simulink model "QuadCopter_Blocks"  (R2014b)
settings: Solver=ode45  StartTime=0.0  StopTime=10.0  RelTol=1e-3
settings Model: Creator=Samy.Amin  LastModifiedBy=Samy.Amin

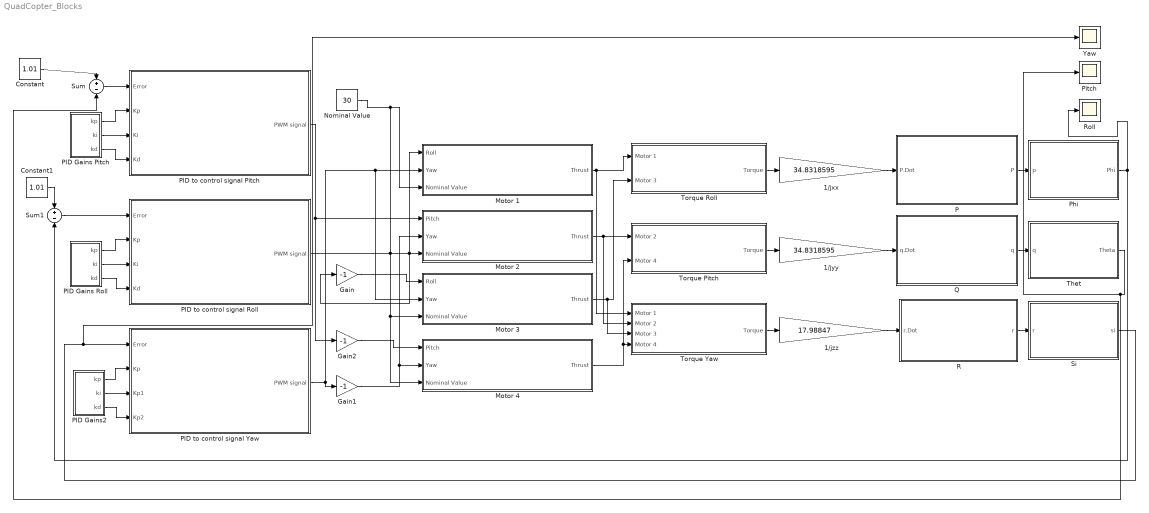
== system QuadCopter_Blocks ==
  1/jxx : Gain  Gain=34.8318595
  1/jyy : Gain  Gain=34.8318595
  1/jzz : Gain  Gain=17.98847
  Constant : Constant  Value=1.01
  Constant1 : Constant  Value=1.01
  Gain : Gain  Gain=-1
  Gain1 : Gain  Gain=-1
  Gain2 : Gain  Gain=-1
  Motor 1 : Subsystem
  Motor 2 : Subsystem
  Motor 3 : Subsystem
  Motor 4 : Subsystem
  Nominal Value : Constant  Value=30
  "P " : Subsystem
  PID Gains Pitch : Subsystem
  PID Gains Roll : Subsystem
  PID Gains2 : Subsystem
  "PID to control signal Pitch " : Subsystem
  PID to control signal Roll : Subsystem
  PID to control signal Yaw : Subsystem
  Phi : Subsystem
  Pitch : Scope
  Q : Subsystem
  R : Subsystem
  Roll : Scope
  Si : Subsystem
  Sum : Sum  Inputs=+-
  Sum1 : Sum  Inputs=+-
  Thet : Subsystem
  Torque Pitch : Subsystem
  Torque Roll : Subsystem
  Torque Yaw : Subsystem
  Yaw : Scope
      settings: SaveName=ScopeData2
  wires:
  "PID to control signal Pitch "/1("PWM signal ") -> Motor 2/1(Pitch), Gain2/1
  Gain2/1 -> Motor 4/1(Pitch)
  PID to control signal Roll/1("PWM signal ") -> Motor 1/1(Roll), Gain/1
  Gain/1 -> Motor 3/1(Roll)
  PID to control signal Yaw/1("PWM signal ") -> Gain1/1, Motor 3/2(Yaw), Motor 1/2(Yaw)
  Gain1/1 -> Motor 4/2(Yaw), Motor 2/2(Yaw)
  Nominal Value/1 -> Motor 4/3(Nominal Value), Motor 3/3(Nominal Value), Motor 2/3(Nominal Value), Motor 1/3(Nominal Value)
  Motor 1/1(Thrust) -> Torque Yaw/1(Motor 1), Torque Roll/1(Motor 1)
  Motor 3/1(Thrust) -> Torque Yaw/3(Motor 3), Torque Roll/2(Motor 3)
  Motor 2/1(Thrust) -> Torque Yaw/2("Motor 2 "), Torque Pitch/1(Motor 2)
  Motor 4/1(Thrust) -> Torque Yaw/4(Motor 4), Torque Pitch/2(Motor 4)
  Torque Roll/1(Torque) -> 1/jxx/1
  Torque Pitch/1(Torque) -> 1/jyy/1
  1/jxx/1 -> "P "/1(P.Dot)
  1/jyy/1 -> Q/1(q.Dot)
  "P "/1(P) -> Phi/1(p)
  Q/1(q) -> Thet/1(q)
  Phi/1(Phi) -> Roll/1, Sum1/2
  Thet/1(Theta) -> Sum/2, Pitch/1
  PID Gains Pitch/1(kp) -> "PID to control signal Pitch "/2(Kp)
  PID Gains Pitch/2(ki) -> "PID to control signal Pitch "/3(Ki)
  PID Gains Pitch/3(kd) -> "PID to control signal Pitch "/4(Kd)
  PID Gains Roll/1(kp) -> PID to control signal Roll/2(Kp)
  PID Gains Roll/2(ki) -> PID to control signal Roll/3(Ki)
  PID Gains Roll/3(kd) -> PID to control signal Roll/4(Kd)
  PID Gains2/1(kp) -> PID to control signal Yaw/2(Kp)
  PID Gains2/2(ki) -> PID to control signal Yaw/3(Kp1)
  PID Gains2/3(kd) -> PID to control signal Yaw/4(Kp2)
  Si/1(si) -> Yaw/1, PID to control signal Yaw/1(Error)
  Constant/1 -> Sum/1
  Sum/1 -> "PID to control signal Pitch "/1(Error)
  Constant1/1 -> Sum1/1
  Sum1/1 -> PID to control signal Roll/1(Error)
  Torque Yaw/1(Torque) -> 1/jzz/1
  R/1(r) -> Si/1(r)
  1/jzz/1 -> R/1(r.Dot)

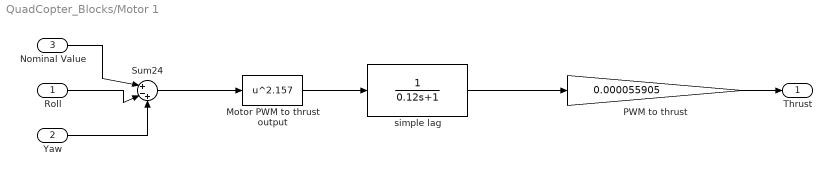
== system QuadCopter_Blocks/Motor 1 ==
  Roll : Inport
  Yaw : Inport  Port=2
  Nominal Value : Inport  Port=3
  Motor PWM to thrust output : Fcn  Expr=u^2.157
  PWM to thrust : Gain  Gain=0.000055905
  Sum24 : Sum  Inputs=|+-+
  simple lag : TransferFcn  Denominator=[0.12 1]
  Thrust : Outport
  wires:
  Roll/1 -> Sum24/2
  Nominal Value/1 -> Sum24/1
  Motor PWM to thrust output/1 -> simple lag/1
  Sum24/1 -> Motor PWM to thrust output/1
  Yaw/1 -> Sum24/3
  simple lag/1 -> PWM to thrust/1
  PWM to thrust/1 -> Thrust/1

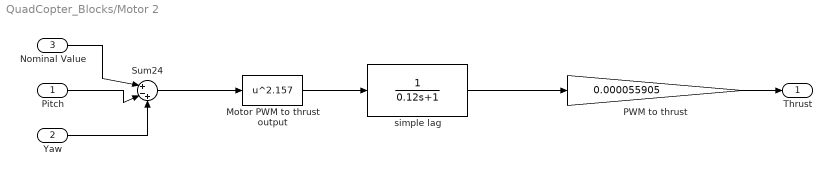
== system QuadCopter_Blocks/Motor 2 ==
  Pitch : Inport
  Yaw : Inport  Port=2
  Nominal Value : Inport  Port=3
  Motor PWM to thrust output : Fcn  Expr=u^2.157
  PWM to thrust : Gain  Gain=0.000055905
  Sum24 : Sum  Inputs=|+-+
  simple lag : TransferFcn  Denominator=[0.12 1]
  Thrust : Outport
  wires:
  Pitch/1 -> Sum24/2
  Nominal Value/1 -> Sum24/1
  Motor PWM to thrust output/1 -> simple lag/1
  Sum24/1 -> Motor PWM to thrust output/1
  Yaw/1 -> Sum24/3
  simple lag/1 -> PWM to thrust/1
  PWM to thrust/1 -> Thrust/1

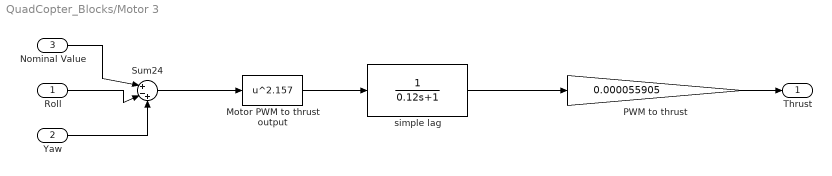
== system QuadCopter_Blocks/Motor 3 ==
  Roll : Inport
  Yaw : Inport  Port=2
  Nominal Value : Inport  Port=3
  Motor PWM to thrust output : Fcn  Expr=u^2.157
  PWM to thrust : Gain  Gain=0.000055905
  Sum24 : Sum  Inputs=|+-+
  simple lag : TransferFcn  Denominator=[0.12 1]
  Thrust : Outport
  wires:
  Roll/1 -> Sum24/2
  Nominal Value/1 -> Sum24/1
  Motor PWM to thrust output/1 -> simple lag/1
  Sum24/1 -> Motor PWM to thrust output/1
  Yaw/1 -> Sum24/3
  simple lag/1 -> PWM to thrust/1
  PWM to thrust/1 -> Thrust/1

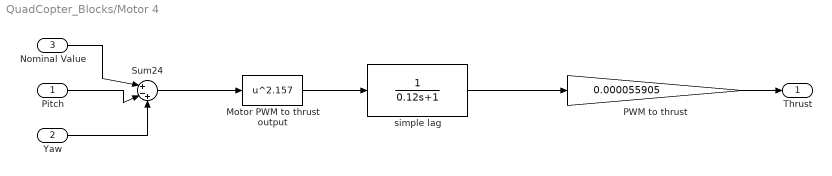
== system QuadCopter_Blocks/Motor 4 ==
  Pitch : Inport
  Yaw : Inport  Port=2
  Nominal Value : Inport  Port=3
  Motor PWM to thrust output : Fcn  Expr=u^2.157
  PWM to thrust : Gain  Gain=0.000055905
  Sum24 : Sum  Inputs=|+-+
  simple lag : TransferFcn  Denominator=[0.12 1]
  Thrust : Outport
  wires:
  Pitch/1 -> Sum24/2
  Nominal Value/1 -> Sum24/1
  Motor PWM to thrust output/1 -> simple lag/1
  Sum24/1 -> Motor PWM to thrust output/1
  Yaw/1 -> Sum24/3
  simple lag/1 -> PWM to thrust/1
  PWM to thrust/1 -> Thrust/1

== system QuadCopter_Blocks/P  ==
  P.Dot : Inport
  rad to degree : Gain  Gain=57.29577951
  simple lag : TransferFcn  Numerator=[0.8]  Denominator=[0.0075 1]
  torque to Phi dot - Jx : TransferFcn  Denominator=[1 0]
  P : Outport
  wires:
  P.Dot/1 -> simple lag/1
  torque to Phi dot - Jx/1 -> rad to degree/1
  simple lag/1 -> torque to Phi dot - Jx/1
  rad to degree/1 -> P/1

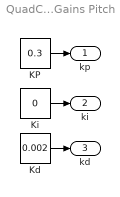
== system QuadCopter_Blocks/PID Gains Pitch ==
  KP : Constant  Value=0.3
  Kd : Constant  Value=0.002
  Ki : Constant  Value=0
  kp : Outport
  ki : Outport  Port=2
  kd : Outport  Port=3
  wires:
  Kd/1 -> kd/1
  KP/1 -> kp/1
  Ki/1 -> ki/1

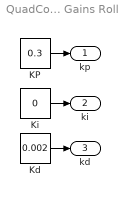
== system QuadCopter_Blocks/PID Gains Roll ==
  KP : Constant  Value=0.3
  Kd : Constant  Value=0.002
  Ki : Constant  Value=0
  kp : Outport
  ki : Outport  Port=2
  kd : Outport  Port=3
  wires:
  Ki/1 -> ki/1
  KP/1 -> kp/1
  Kd/1 -> kd/1

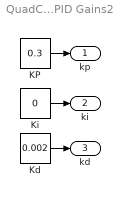
== system QuadCopter_Blocks/PID Gains2 ==
  KP : Constant  Value=0.3
  Kd : Constant  Value=0.002
  Ki : Constant  Value=0
  kp : Outport
  ki : Outport  Port=2
  kd : Outport  Port=3
  wires:
  Kd/1 -> kd/1
  KP/1 -> kp/1
  Ki/1 -> ki/1

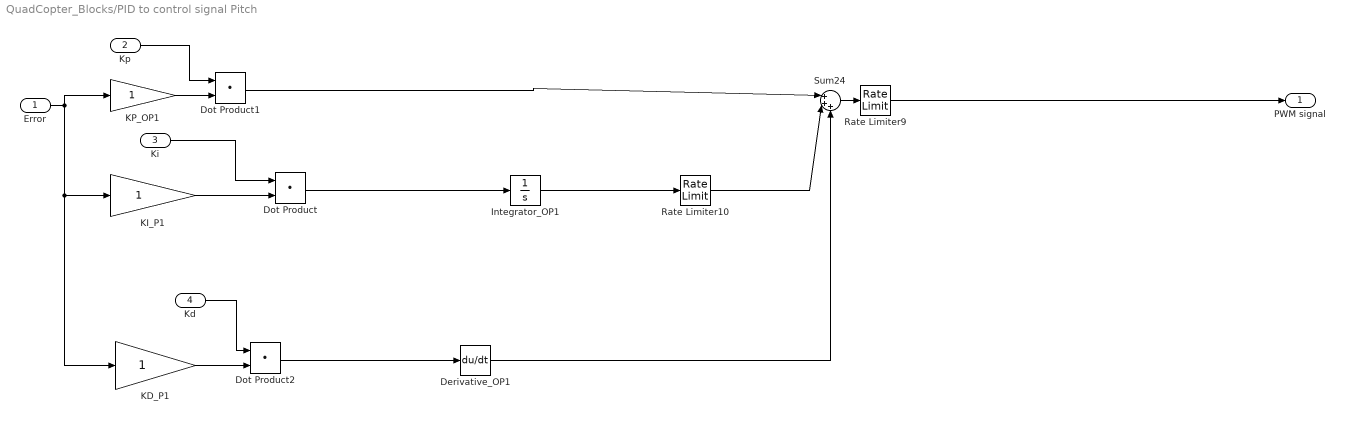
== system QuadCopter_Blocks/PID to control signal Pitch  ==
  Error : Inport
  Kp : Inport  Port=2
  Ki : Inport  Port=3
  Kd : Inport  Port=4
  Derivative_OP1 : Derivative
  Dot Product : DotProduct  InputSameDT=on  OutDataTypeStr=Inherit: Inherit via internal rule
  Dot Product1 : DotProduct  InputSameDT=on  OutDataTypeStr=Inherit: Inherit via internal rule
  Dot Product2 : DotProduct  InputSameDT=on  OutDataTypeStr=Inherit: Inherit via internal rule
  Integrator_OP1 : Integrator
  KD_P1 : Gain
  KI_P1 : Gain
  KP_OP1 : Gain
  Rate Limiter10 : RateLimiter  RisingSlewLimit=399  FallingSlewLimit=-399  SampleTimeMode=inherited
  Rate Limiter9 : RateLimiter  RisingSlewLimit=551  FallingSlewLimit=-551  SampleTimeMode=inherited
  Sum24 : Sum  Inputs=|+++
  "PWM signal " : Outport
  wires:
  Rate Limiter10/1 -> Sum24/2
  Error/1 -> KD_P1/1, KI_P1/1, KP_OP1/1
  Derivative_OP1/1 -> Sum24/3
  Integrator_OP1/1 -> Rate Limiter10/1
  Rate Limiter9/1 -> "PWM signal "/1
  Sum24/1 -> Rate Limiter9/1
  Kp/1 -> Dot Product1/1
  KP_OP1/1 -> Dot Product1/2
  Dot Product1/1 -> Sum24/1
  Ki/1 -> Dot Product/1
  KI_P1/1 -> Dot Product/2
  Dot Product/1 -> Integrator_OP1/1
  Kd/1 -> Dot Product2/1
  KD_P1/1 -> Dot Product2/2
  Dot Product2/1 -> Derivative_OP1/1

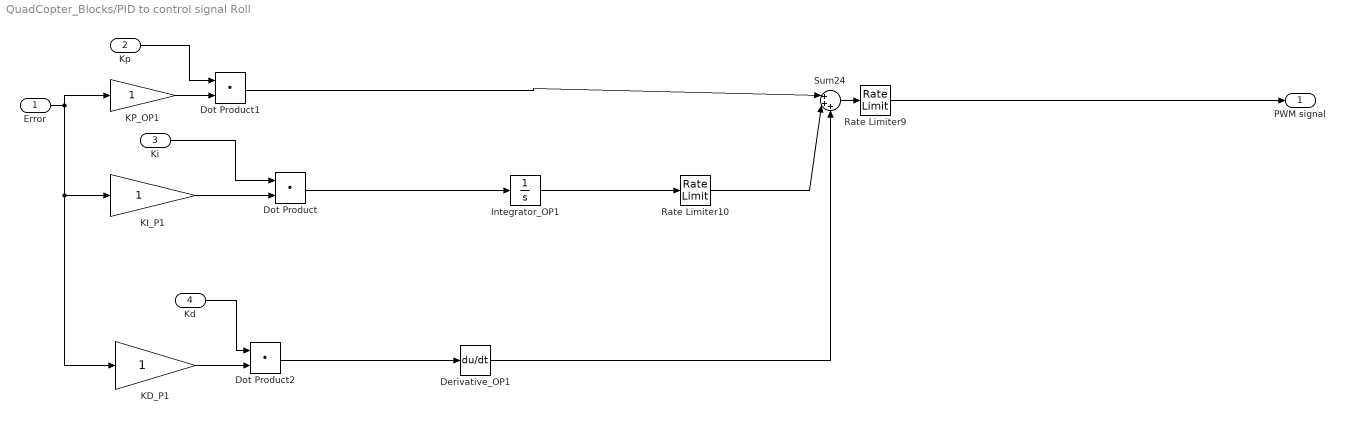
== system QuadCopter_Blocks/PID to control signal Roll ==
  Error : Inport
  Kp : Inport  Port=2
  Ki : Inport  Port=3
  Kd : Inport  Port=4
  Derivative_OP1 : Derivative
  Dot Product : DotProduct  InputSameDT=on  OutDataTypeStr=Inherit: Inherit via internal rule
  Dot Product1 : DotProduct  InputSameDT=on  OutDataTypeStr=Inherit: Inherit via internal rule
  Dot Product2 : DotProduct  InputSameDT=on  OutDataTypeStr=Inherit: Inherit via internal rule
  Integrator_OP1 : Integrator
  KD_P1 : Gain
  KI_P1 : Gain
  KP_OP1 : Gain
  Rate Limiter10 : RateLimiter  RisingSlewLimit=399  FallingSlewLimit=-399  SampleTimeMode=inherited
  Rate Limiter9 : RateLimiter  RisingSlewLimit=551  FallingSlewLimit=-551  SampleTimeMode=inherited
  Sum24 : Sum  Inputs=|+++
  "PWM signal " : Outport
  wires:
  Rate Limiter10/1 -> Sum24/2
  Error/1 -> KD_P1/1, KI_P1/1, KP_OP1/1
  Derivative_OP1/1 -> Sum24/3
  Integrator_OP1/1 -> Rate Limiter10/1
  Rate Limiter9/1 -> "PWM signal "/1
  Sum24/1 -> Rate Limiter9/1
  Kp/1 -> Dot Product1/1
  KP_OP1/1 -> Dot Product1/2
  Dot Product1/1 -> Sum24/1
  Ki/1 -> Dot Product/1
  KI_P1/1 -> Dot Product/2
  Dot Product/1 -> Integrator_OP1/1
  Kd/1 -> Dot Product2/1
  KD_P1/1 -> Dot Product2/2
  Dot Product2/1 -> Derivative_OP1/1

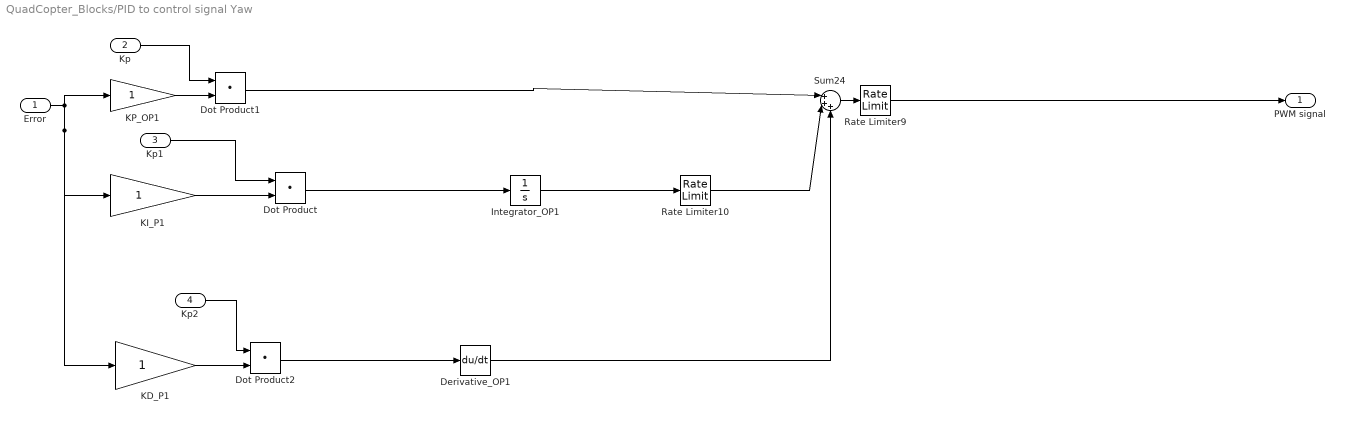
== system QuadCopter_Blocks/PID to control signal Yaw ==
  Error : Inport
  Kp : Inport  Port=2
  Kp1 : Inport  Port=3
  Kp2 : Inport  Port=4
  Derivative_OP1 : Derivative
  Dot Product : DotProduct  InputSameDT=on  OutDataTypeStr=Inherit: Inherit via internal rule
  Dot Product1 : DotProduct  InputSameDT=on  OutDataTypeStr=Inherit: Inherit via internal rule
  Dot Product2 : DotProduct  InputSameDT=on  OutDataTypeStr=Inherit: Inherit via internal rule
  Integrator_OP1 : Integrator
  KD_P1 : Gain
  KI_P1 : Gain
  KP_OP1 : Gain
  Rate Limiter10 : RateLimiter  RisingSlewLimit=399  FallingSlewLimit=-399  SampleTimeMode=inherited
  Rate Limiter9 : RateLimiter  RisingSlewLimit=551  FallingSlewLimit=-551  SampleTimeMode=inherited
  Sum24 : Sum  Inputs=|+++
  "PWM signal " : Outport
  wires:
  Rate Limiter10/1 -> Sum24/2
  Error/1 -> KD_P1/1, KI_P1/1, KP_OP1/1
  Derivative_OP1/1 -> Sum24/3
  Integrator_OP1/1 -> Rate Limiter10/1
  Rate Limiter9/1 -> "PWM signal "/1
  Sum24/1 -> Rate Limiter9/1
  Kp/1 -> Dot Product1/1
  KP_OP1/1 -> Dot Product1/2
  Dot Product1/1 -> Sum24/1
  Kp1/1 -> Dot Product/1
  KI_P1/1 -> Dot Product/2
  Dot Product/1 -> Integrator_OP1/1
  Kp2/1 -> Dot Product2/1
  KD_P1/1 -> Dot Product2/2
  Dot Product2/1 -> Derivative_OP1/1

== system QuadCopter_Blocks/Phi ==
  p : Inport
  angle dot to angle : TransferFcn  Denominator=[1 0]
  Phi : Outport
  wires:
  p/1 -> angle dot to angle/1
  angle dot to angle/1 -> Phi/1

== system QuadCopter_Blocks/Q ==
  q.Dot : Inport
  rad to degree : Gain  Gain=57.29577951
  simple lag : TransferFcn  Numerator=[0.8]  Denominator=[0.0075 1]
  torque to Phi dot - Jx : TransferFcn  Denominator=[1 0]
  q : Outport
  wires:
  rad to degree/1 -> q/1
  simple lag/1 -> torque to Phi dot - Jx/1
  torque to Phi dot - Jx/1 -> rad to degree/1
  q.Dot/1 -> simple lag/1

== system QuadCopter_Blocks/R ==
  r.Dot : Inport
  rad to degree : Gain  Gain=57.29577951
  simple lag : TransferFcn  Numerator=[0.8]  Denominator=[0.0075 1]
  torque to Phi dot - Jx : TransferFcn  Denominator=[1 0]
  r : Outport
  wires:
  r.Dot/1 -> simple lag/1
  torque to Phi dot - Jx/1 -> rad to degree/1
  simple lag/1 -> torque to Phi dot - Jx/1
  rad to degree/1 -> r/1

== system QuadCopter_Blocks/Si ==
  r : Inport
  angle dot to angle : TransferFcn  Denominator=[1 0]
  si : Outport
  wires:
  r/1 -> angle dot to angle/1
  angle dot to angle/1 -> si/1

== system QuadCopter_Blocks/Thet ==
  q : Inport
  angle dot to angle : TransferFcn  Denominator=[1 0]
  Theta : Outport
  wires:
  angle dot to angle/1 -> Theta/1
  q/1 -> angle dot to angle/1

== system QuadCopter_Blocks/Torque Pitch ==
  Motor 2 : Inport
  Motor 4 : Inport  Port=2
  Length : Gain  Gain=0.34
  Sum1 : Sum  Inputs=|+-
  Torque : Outport
  wires:
  Sum1/1 -> Length/1
  Motor 2/1 -> Sum1/1
  Length/1 -> Torque/1
  Motor 4/1 -> Sum1/2

== system QuadCopter_Blocks/Torque Roll ==
  Motor 1 : Inport
  Motor 3 : Inport  Port=2
  Length : Gain  Gain=0.34
  Sum1 : Sum  Inputs=|+-
  Torque : Outport
  wires:
  Sum1/1 -> Length/1
  Motor 1/1 -> Sum1/1
  Length/1 -> Torque/1
  Motor 3/1 -> Sum1/2

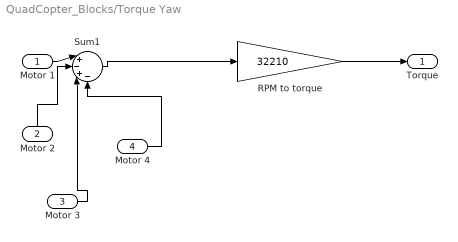
== system QuadCopter_Blocks/Torque Yaw ==
  Motor 1 : Inport
  "Motor 2 " : Inport  Port=2
  Motor 3 : Inport  Port=3
  Motor 4 : Inport  Port=4
  "RPM to torque " : Gain  Gain=32210
  Sum1 : Sum  Inputs=|+-+-
  Torque : Outport
  wires:
  "Motor 2 "/1 -> Sum1/2
  "RPM to torque "/1 -> Torque/1
  Motor 1/1 -> Sum1/1
  Sum1/1 -> "RPM to torque "/1
  Motor 3/1 -> Sum1/3
  Motor 4/1 -> Sum1/4
